simulink model "Team7_Final_Simulink_Model"  (R2024a)
settings: Solver=VariableStepAuto  StartTime=0.0  StopTime=20  RelTol=1e-3
libraries: simulink x2, commcnvcod2 x2, commdigbbndpm3 x2, commfilt2 x2, dspquant2 x2, commchan3 x1, dspsnks4 x1, commsink2 x1, dspvision x1
settings Model: LastModifiedBy=sakshammahajan

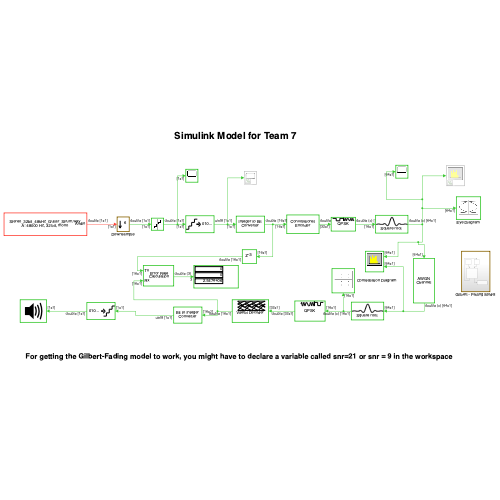
[thumbnail: Simulink's stored preview of the top-level diagram]
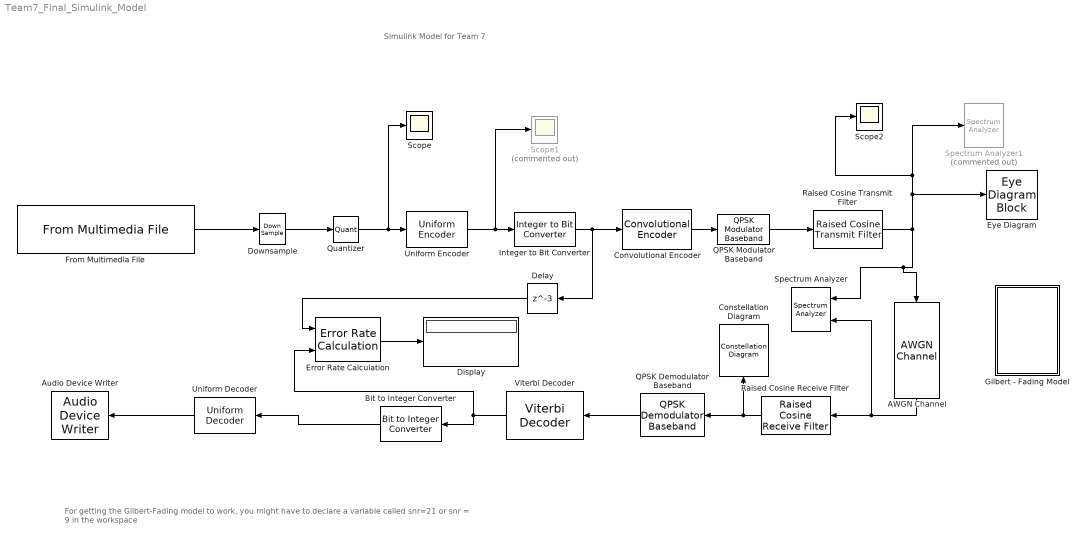
== system Team7_Final_Simulink_Model ==
  note: Simulink Model for Team 7
  note: For getting the Gilbert-Fading model to work, you might have to declare a variable called snr=21 or snr = 9 in the workspace
  AWGN Channel : commchan3/AWGN Channel  LegacyMode=off  NoiseMethod="Signal to noise ratio  (SNR)"  noiseMode="Signal to noise ratio  (SNR)"  EbNo=10  EsNo=10  SNR=snr  BitsPerSymbol=1  SignalPower=1  SamplesPerSymbol=1  SymbolPeriod=1  VarianceSource=Parameter  Variance=1  RandomStream=Global stream  Seed=5  SimulateUsing=Code generation
  Audio Device Writer : dspsnks4/Audio Device Writer  Driver=CoreAudio  Device=Default  InheritSampleRate=on  SampleRate=44100  BitDepth=16-bit integer  BufferSize=4096  NumBuffers=10  DefaultOutputChannelMapping=on  OutputChannelMapping=1:2  OutputNumUnderrunSamples=off  DriverIdx=5  DeviceWarnFlag=''
  Bit to Integer Converter : simulink/Logic and Bit Operations/Bit to Integer Converter  nbits=16  bitOrder=MSB first  signedOutputValues=Unsigned  outDtype=uint8  outDtypeSigned=Inherit via internal rule
  Constellation Diagram : ConstellationDiagram  WindowPosition=[10.000000,66.000000,600.000000,600.000000,]  ScopeFrameLocation=window  DefaultConfigurationName=comm.scopes.ConstellationDiagramBlockCfg
  Convolutional Encoder : commcnvcod2/Convolutional Encoder  trellis=poly2trellis(7, [171 133])  opMode=Continuous  DelayedResetAction=on  hasIniStPort=off  hasFinStPort=off  usePuncVector=off  punctureVector=[1; 1; 0; 1; 0; 1]  reset=Unused parameter value
      settings: LibrarySourceBlock=|
      | commhdlcnvcod/Convolutional
      | Encoder
  Delay : Delay  DelayLength=3  InitialCondition=0
  Display : Display
  Downsample : DownSample  N=6  RateOptions=Allow multirate processing
  Error Rate Calculation : commsink2/Error Rate Calculation  N=0  st_delay=48  cp_mode=Entire frame  subframe=[]  PMode=Port  WsName=ErrorVec  RsMode2=off  stop=off  numErr=100  maxBits=1e6
  Eye Diagram : EyeDiagramBlock  WindowPosition=[641.000000,120.000000,800.000000,500.000000,]  ScopeFrameLocation=window
  From Multimedia File : dspvision/From Multimedia File  inputFilename=/Users/sakshammahajan/Desktop/ELEC391/ELEC391_Sound_Files/Stereo_32bit_48kHz_Guitar_Strum.wav  readRange=[1 Inf]  loop=on  numPlays=inf  outputStreams=Audio only  videoDataType=single  audioDataType=double  inheritSampleTime=on  userDefinedSampleTime=1/30  noAudioOutput=off  isIntensityVideo=off  fourcc=RGB  colorVideoFormat=Separate color signals  outputEOF=off  dataOrg=Column-major  audioFrameSize=1  computeAudioFrameSize=off  outSamplingMode=Sample based
      settings: LibrarySourceBlock=audiosources/From Multimedia File
  Gilbert - Fading Model : Subsystem
  Integer to Bit Converter : simulink/Logic and Bit Operations/Integer to Bit Converter  nbits=16  signedInputValues=Unsigned  bitOrder=MSB first  outDtype=double
  QPSK Demodulator Baseband : commdigbbndpm3/QPSK Demodulator Baseband  OutType=Bit  DecType=Hard decision  VarSource=Dialog  Variance=1  Dec=Gray  Ph=pi/4  outDtype1=Inherit via internal rule  outDtype2=Inherit via internal rule  derotateFactorWordLen=16  derotateFactorDataTypeStr=Inherit: Same word length as input  derotateFactorLastDataTypeStr=Inherit: Same word length as input
      settings: LibrarySourceBlock=|
      | commhdldigbbndpm/QPSK
      | Demodulator
      | Baseband
  QPSK Modulator Baseband : commdigbbndpm3/QPSK Modulator Baseband  InType=Bit  Enc=Gray  Ph=pi/4  outDtype=double  outWordLen=16  outUDDataType=sfix(16)  outFracLenMode=Best precision  outFracLen=15  outDataTypeStr=double  outLastDataTypeStr=double
      settings: LibrarySourceBlock=|
      | commhdldigbbndpm/QPSK
      | Modulator
      | Baseband
  Quantizer : Quantizer  QuantizationInterval=0.0625
  Raised Cosine Receive Filter : commfilt2/Raised Cosine Receive Filter  filtType=Square root  R=0.3  filtSpan=16  N=4  downFactor=4  downOffset=0  filterGain=1  InputProcessing=Columns as channels (frame based)  RateOptions=Enforce single-rate processing  framing=Mute  checkCoeff=off  variableName=rcRxFilt  currentFiltSpan=10  D=5  inputOffset=0  sampMode=Mute  saveAsFlag=0  rateMode=Downsampling  checkGain=Normalized  launchFVT=on  roundingMode=Floor  overflowMode=off  coeffDataTypeStr=Inherit: Same word length as input  coeffMin=[]  coeffMax=[]  coeffLastDataTypeStr=Inherit: Same word length as input  accumDataTypeStr=Inherit: Same as product output  accumLastDataTypeStr=Inherit: Same as product output  outputDataTypeStr=Inherit: Same as accumulator  outputMin=[]  outputMax=[]  outputLastDataTypeStr=Inherit: Same as accumulator
      settings: LibrarySourceBlock=|
      | commhdlfilt/Raised Cosine
      | Receive Filter
  Raised Cosine Transmit Filter : commfilt2/Raised Cosine Transmit Filter  filtType=Square root  R=0.3  filtSpan=16  N=4  filterGain=1  InputProcessing=Columns as channels (frame based)  RateOptions=Enforce single-rate processing  framing=Mute  checkCoeff=off  variableName=rcTxFilt  checkGain=Normalized  sampMode=Mute  saveAsFlag=0  currentFiltSpan=10  D=5  launchFVT=on  roundingMode=Floor  overflowMode=off  coeffDataTypeStr=Inherit: Same word length as input  coeffMin=[]  coeffMax=[]  coeffLastDataTypeStr=Inherit: Same word length as input  outputDataTypeStr=Inherit: Same as accumulator  outputMin=[]  outputMax=[]  outputLastDataTypeStr=Inherit: Same as accumulator
      settings: LibrarySourceBlock=|
      | commhdlfilt/Raised Cosine
      | Transmit Filter
  Scope : Scope
  Scope1 : Scope  Commented=on
  Scope2 : Scope
  Spectrum Analyzer : SpectrumAnalyzer  NumInputPorts=2  WindowPosition=[266.000000,43.000000,960.000000,623.000000,]  ScopeFrameLocation=window  Span=128000  StartFrequency=-64000  StopFrequency=64000  YLimits=[-112.75255665,27.3826655]  ShowLegend=on  ExpandToolstrip=on  SelectedToolstripTab=spectrumAnalyzerToolstrip.measurementsTab
  Spectrum Analyzer1 : SpectrumAnalyzer  Commented=on  WindowPosition=[279.000000,83.000000,800.000000,500.000000,]  ScopeFrameLocation=window  Span=1024000  StartFrequency=-512000  StopFrequency=512000  YLimits=[-115.66449024,36.4322386]  ExpandToolstrip=on  SelectedToolstripTab=spectrumAnalyzerToolstrip.measurementsTab
  Uniform Decoder : dspquant2/Uniform Decoder  peak=1  bits=8  overflowMode=Saturate  otype=double
  Uniform Encoder : dspquant2/Uniform Encoder  peak=1  bits=8  otype=Unsigned integer
  Viterbi Decoder : commcnvcod2/Viterbi Decoder  trellis=poly2trellis(7, [171 133])  isPunctured=off  punctureVector=[1; 1; 0; 1; 0; 1]  erasures=off  dectype=Hard decision  nsdecb=4  runSigValErrCheck=off  tbdepth=32  opmode=Continuous  reset=off  delayedResetAction=on  smWordLength=16  outDataType=double
      settings: LibrarySourceBlock=commhdlcnvcod/Viterbi Decoder
  wires:
  Downsample/1 -> Quantizer/1
  Quantizer/1 -> Scope/1, Uniform Encoder/1
  Uniform Encoder/1 -> Integer to Bit Converter/1, Scope1/1
  Convolutional Encoder/1 -> QPSK Modulator Baseband/1
  QPSK Demodulator Baseband/1 -> Viterbi Decoder/1
  QPSK Modulator Baseband/1 -> Raised Cosine Transmit Filter/1
  Raised Cosine Receive Filter/1 -> Constellation Diagram/1, QPSK Demodulator Baseband/1
  Raised Cosine Transmit Filter/1 -> Eye Diagram/1, Spectrum Analyzer1/1, Scope2/1, Spectrum Analyzer/1, AWGN Channel/1
  Uniform Decoder/1 -> Audio Device Writer/1
  From Multimedia File/1 -> Downsample/1
  Error Rate Calculation/1 -> Display/1
  Viterbi Decoder/1 -> Error Rate Calculation/2, Bit to Integer Converter/1
  AWGN Channel/1 -> Spectrum Analyzer/2, Raised Cosine Receive Filter/1
  Integer to Bit Converter/1 -> Delay/1, Convolutional Encoder/1
  Bit to Integer Converter/1 -> Uniform Decoder/1
  Delay/1 -> Error Rate Calculation/1

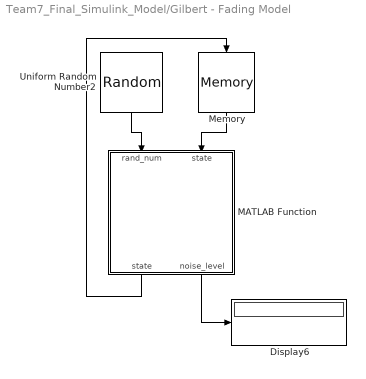
== system Team7_Final_Simulink_Model/Gilbert - Fading Model ==
  Display6 : Display
  MATLAB Function : MATLAB Function  TreatAsAtomicUnit=on
  Memory : Memory  InitialCondition=1  StateName=snr
  Uniform Random Number2 : UniformRandomNumber  Seed=3  SampleTime=0.1
  wires:
  MATLAB Function/2(noise_level) -> Display6/1
  Memory/1 -> MATLAB Function/2("state ")
  Uniform Random Number2/1 -> MATLAB Function/1(rand_num)
  MATLAB Function/1(state) -> Memory/1

== matlab function Team7_Final_Simulink_Model/Gilbert - Fading Model/MATLAB Function ==
  data: rand_num input; state output; state input; noise_level output
function [state, noise_level] = gilbert_fading(rand_num, state)%inputs are rand_num, state. Outputs are state, noise_level
    % Transition probabilities
    P_good_to_bad = 0.07;
    P_bad_to_good = 0.15;
    snr = 21;

    % Noise levels
    snr_good = 21; % snr in Good state
    snr_bad = 9;  % snr in Bad state

    switch state
        case 1 % Good state
            if rand_num < P_good_to_bad
                state = 0; % Transition to Bad state
            end
            noise_level = snr_good;
            assignin('base','snr',21); % set value of snr to 21 
            %snr = 21;
        case 0 % Bad state
            if rand_num < P_bad_to_good
                state = 1; % Transition to Good state
            end
            noise_level = snr_bad;
            %snr = 9;
            assignin('base','snr',9); % set value of snr to 9
        otherwise
            state = 1; % Default to Good state
            noise_level = snr_good;
            %snr = 21;
            assignin('base','snr',21); % set value of snr to 21
    end
end
